simulink model "Main"  (R2022a)
settings: Solver=VariableStepAuto  StartTime=0.0  StopTime=30  RelTol=1e-3
values from neighbouring files (symbols this model uses):
  A_eq = double(A_eq)    [source_export.m]
  b = 7.66e-5    (= 7.66e-05)    [source_export.m]
  B_eq = double(B_eq)    [source_export.m]
  C = [1 0 0 0 0 0 0 0 0 0 0 0 ... (first row only)    [source_export.m]
  C_eq = C_final([1 2 3 6], 1:12)    [source_export.m]
  C_simulink = eye(12)    [source_export.m]
  Condition_0 = transpose([0 0 0 0 0 0 0 0 0 0 0 0])    [source_export.m]
  Condition_1 = transpose([0.2 0.2 0.2 0.2 0.2 0.2 0.2 0.2 0.2 0.2 0.2 0.2])    [source_export.m]
  D = zeros(4,4)    [source_export.m]
  d = 5.63e-6    (= 5.63e-06)    [source_export.m]
  D_Simulink = zeros(12,4)    [source_export.m]
  F = [      -20,   -20,   -20,   -21,   -21,   15,   -21.5, -21.5 ... (first row only)    [source_export.m]
  g = 9.81    [source_export.m]
  inv_G0 = inv_G_0( : , [1 , 2 ,3 ,6])    [source_export.m]
  inv_G0_LQR = inv_G_0_LQR( : , [1 , 2 ,3 ,6])    [source_export.m]
  Ixx = 8.5532e-3    (= 0.0085532)    [source_export.m]
  Iyy = 8.5532e-3    (= 0.0085532)    [source_export.m]
  Izz = 1.476e-2    (= 0.01476)    [source_export.m]
  K_d_LQR = K_LQR(:,1:12)    [source_export.m]
  K_q_LQR = K_LQR(:,12+1:12+4)    [source_export.m]
  Kfeedback = place(A_eq,B_eq,Poles)    [source_export.m]
  L = place(A_eq.',C_eq.',poles_obsv).'    [source_export.m]
  l = 0.22    [source_export.m]
  L_RO = 100*[1 2 1 14 ... (first row only)    [source_export.m]
  m = 1    [source_export.m]
  Q_1 = inv_mat2(:,1:q)    [source_export.m]
  Q_2 = inv_mat2(:,q+1:n)    [source_export.m]
  T_O = lyap(-F,A_eq,-L_RO*C)    [source_export.m]
undefined symbols (not defined in the file or in its folder): Discrete, K_LQR1, Time
libraries: slpidlib x8, simulink x6, ctrlSharedLib x1, sim3dlib x1, uavsim3dlib x1
(part 1 of 2)
settings Model: Creator=ali14  LastModifiedBy=ali14
settings ModelReferenceCC: EnableRefExpFcnMdlSchedulingChecks=off
settings RTWCC: Description=Generic Real-Time Target

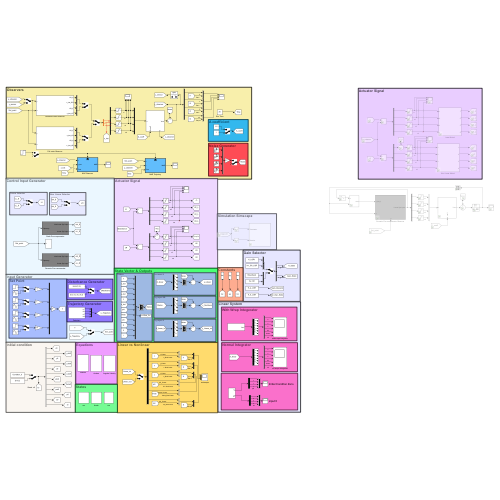
[thumbnail: Simulink's stored preview of the top-level diagram]
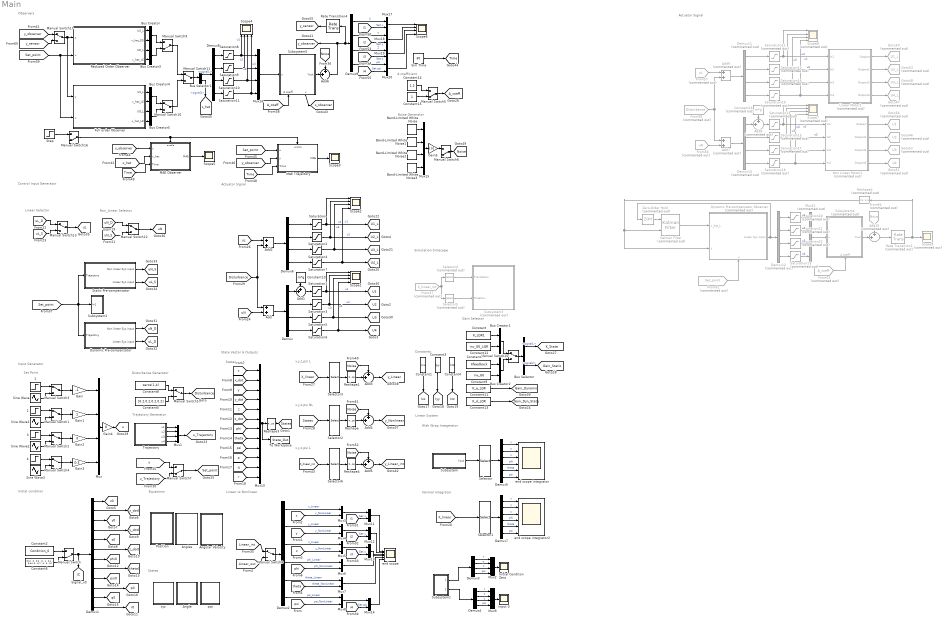
== system Main ==
  note: Observers
  note: A coefficient
  note: Noise Generator
  note: Gain Selector
  note: Actuator Signal
  note: States
  note: x,y,z,psi NL
  note: x,y,z,psi L
  note: Normal Integrator
  note: Trajectory Generator
  note: Linear Selector
  note: Non_Linear Selector
  note: Set Point
  note: Disturbance Generator
  note: State Vector & Outputs
  note: With Wrap Integerator
  note: Linear System
  note: Linear vs Nonlinear
  note: Constants
  note: Initial condition
  note: States
  note: Equations
  note: Input Generator
  note: Control Input Generator
  note: x,y,z,psi L
  note: Simulation Simscape
  note: Actuator Signal
  1 : Step  Time=3  SampleTime=0
  2 : Step  Time=3  SampleTime=0
  3 : Step  Time=0  SampleTime=0
  4 : Step  Time=5  SampleTime=0
  Add : Sum
  Add{1,3..6} (5 alike) : Sum  Inputs=++|
  Add10 : Sum  Commented=on  Inputs=++|
  Add2 : Sum
  Add7 : Sum  Commented=on
  Add8 : Sum  Commented=on  Inputs=++|
  Add9 : Sum  Commented=on
  Angle : Subsystem
  Angles : Subsystem
  Angular Velocity : Subsystem
  Band-Limited White Noise : simulink/Sources/Band-Limited White Noise  Cov=[0.000001]  Ts=0.01  seed=[23341]
  Band-Limited White Noise1 : simulink/Sources/Band-Limited White Noise  Cov=[0.000001]  Ts=0.1  seed=[23341]
  Band-Limited White Noise2 : simulink/Sources/Band-Limited White Noise  Cov=[0.0001]  Ts=0.1  seed=[23341]
  Band-Limited White Noise3 : simulink/Sources/Band-Limited White Noise  Cov=[0.00001]  Ts=0.1  seed=[23341]
  Bus Creator{,1..5} (6 alike) : BusCreator  Inputs=2
  Bus Selector : BusSelector  OutputSignals=signal1,signal2
  Bus Selector1 : BusSelector  OutputSignals=signal1,signal2
  Constant : Constant  Value=K_LQR1
  Constant1 : Constant  Value=Ixx
  Constant10 : Constant  Value=m*g
  Constant11 : Constant  Value=K_q_LQR
  Constant12 : Constant  Value=inv_G0_LQR
  Constant13 : Constant  Value=K_d_LQR
  Constant14 : Constant  Value=1.2
  Constant15 : Constant
  Constant16 : Constant  Commented=on  Value=m*g
  Constant2 : Constant  Value=Condition_0
  Constant3 : Constant  Value=Iyy
  Constant4 : Constant  Value=Izz
  Constant5 : Constant  Value=[0.2,0.2,0.2,0.2]
  Constant6 : Constant  Value=[0.2 , 0 , 0.2 , 0 , 1 , 0.4 , 0.04 ,0 , 0.7 , 0 , 0 , 0]
  Constant7 : Constant  Value=Kfeedback
  Constant8 : Constant  Value=zeros(1,4)
  Constant9 : Constant  Value=inv_G0
  Demux{,3..4,6,8..9} (6 alike) : Demux
  Demux1 : Demux  Outputs=12
  Demux10 : Demux  Commented=on
  Demux11 : Demux  Commented=on
  Demux12 : Demux  Commented=on
  Demux2 : Demux  Outputs=6
  Demux5 : Demux  Outputs=6
  Demux7 : Demux  Outputs=6
  Dynamic Pre-compensator : Subsystem
  Dynamic Pre-compensator Observer : Subsystem  Commented=on
      settings: PortSchema="{\"entries\":[{\"content\":{\"sides\":[{\"content\":{\"connectorIds\":[\"In1\",\"In2\"]},\"type\":\"ConnectorPlacement.EquallySpacedRectSide\",\"uuid\":\"7ff58fb8-8d2b-4c8e-a591-1a745530a661\"},{\"content\":{\"connectorIds\":[\"Out1\"],\"side\":\"RIGHT\"},\"type\":\"ConnectorPlacement.EquallySpacedRectSide\",\"uuid\":\"18d93ec8-0d87-4739-af88-4b64d8e2703a\"},{\"content\":{\"connectorIds\":[],\"side\":\"TOP\"},\"type\":\"ConnectorPlacement.EquallySpacedRectSide\",\"uuid\":\"fcb1c7ab-ae0a-4067-b3dc-1c5dc69aae1f\"},{\"content\":{\"connectorIds\":[\"In3\"],\"side\":\"BOTTOM\"},\"type\":\"ConnectorPlacement.EquallySpacedRectSide\",\"uuid\":\"838d79c5-32f8-45c9-a35f-55d5e51129e3\"}]},\"type\":\"ConnectorPlacement.EquallySpacedConnector\",\"uuid\":\"97c2476e-220b-403a-9339-6beb5ac026c2\"}],\"packageUris\":[\"http://schema.mathworks.com/mf0/Connector/R2020b\"],\"version\":\"1.0\"}"
  From47 : From  Commented=on  GotoTag=X_linear_int  TagVisibility=global
  From56 : From  Commented=on  GotoTag=uN  TagVisibility=global
  From57 : From  Commented=on  GotoTag=uL  TagVisibility=global
  From58 : From  Commented=on  GotoTag=Disturbance  TagVisibility=global
  From62 : From  Commented=on  GotoTag=Set_point  TagVisibility=global
  From63 : From  Commented=on  GotoTag=A_coeff  TagVisibility=global
  From64 : From  Commented=on  GotoTag=Noise  TagVisibility=global
  Full order Observer : Subsystem
  Gain : Gain  Gain=-1
  Gain1 : Gain
  Gain2 : Gain  Gain=3
  Gain3 : Gain  Gain=0.3
  Gain4 : Gain  Gain=0
  Gain5 : Gain  Gain=0.01
  Goto46 : Goto  Commented=on  GotoTag=U2  TagVisibility=global
  Goto47 : Goto  Commented=on  GotoTag=U4_L  TagVisibility=global
  Goto48 : Goto  Commented=on  GotoTag=U3_L  TagVisibility=global
  Goto50 : Goto  Commented=on  GotoTag=U1_L  TagVisibility=global
  Goto51 : Goto  Commented=on  GotoTag=U4  TagVisibility=global
  Goto52 : Goto  Commented=on  GotoTag=U3  TagVisibility=global
  Goto53 : Goto  Commented=on  GotoTag=U2_L  TagVisibility=global
  Goto54 : Goto  Commented=on  GotoTag=U1  TagVisibility=global
  Initial Conditon Zero : Scope
  Kalman Filter : ctrlSharedLib/Kalman Filter  Commented=on  TimeDomain=Discrete-Time  UseCurrentEstimator=on  ModelSource=Individual A, B, C, D matrices  ModelSourceVariable=ss(0.95,1,1,0,1)  A=A_eq  B=B_eq  C=C_eq  D=D  NumberOfStates=12  NumberOfInputs=4  NumberOfOutputs=4  InitialEstimateSource=Dialog  X0=0  P0=10  UseK=off  UseGH=off  NumberOfProcessNoiseInputs=1  G=1  TimeInvariantG=on  H=0  TimeInvariantH=on  Q=0.05  TimeInvariantQ=on  R=1  TimeInvariantR=on  N=0  TimeInvariantN=on  AddInputPort=on  AddEnablePort=off  OutputEstimatedY=off  OutputP=off  Ts=-1
  Linear Motor1 : Subsystem  Commented=on
  MAE Observer : Subsystem
  MAE Trajectory : Subsystem
  Manual Switch{,5..7,9,16} (6 alike) : ManualSwitch  CurrentSetting=0
  Manual Switch{1..4,8,10..15,17} (12 alike) : ManualSwitch
  Mux{,1..2,9,15..16} (6 alike) : Mux
  Mux10 : Mux  Inputs=12
  Mux{3..8,11..14,17..20} (14 alike) : Mux  Inputs=2
  Mux21 : Mux  Commented=on
  Non Linear Motor1 : Subsystem  Commented=on
  Position : Subsystem
  Rate Transition1 : RateTransition  Commented=on  OutPortSampleTime=0.01
  Rate Transition4 : RateTransition  OutPortSampleTime=0.01
  Reduced Order Observer : Subsystem
  Reshape{,1,3..4} (4 alike) : Reshape  OutputDimensionality=Column vector (2-D)
  Reshape2 : Reshape  Commented=on  OutputDimensionality=Column vector (2-D)
  Saturation : Saturate  UpperLimit=15  LowerLimit=-10
  Saturation1 : Saturate  UpperLimit=25  LowerLimit=0
  Saturation{2..5,9..10} (6 alike) : Saturate  UpperLimit=1.5  LowerLimit=-1.5
  Saturation11 : Saturate  UpperLimit=1  LowerLimit=-1
  Saturation12 : Saturate  Commented=on  UpperLimit=15  LowerLimit=-10
  Saturation13 : Saturate  Commented=on  UpperLimit=25  LowerLimit=0
  Saturation{14..17,21..22} (6 alike) : Saturate  Commented=on  UpperLimit=1.5  LowerLimit=-1.5
  Saturation18 : Saturate  Commented=on  UpperLimit=1  LowerLimit=-1
  Saturation19 : Saturate  Commented=on  UpperLimit=1  LowerLimit=-1
  Saturation20 : Saturate  Commented=on  UpperLimit=15  LowerLimit=-10
  Saturation23 : Saturate  Commented=on  UpperLimit=1  LowerLimit=-1
  Saturation6 : Saturate  UpperLimit=1  LowerLimit=-1
  Saturation7 : Saturate  UpperLimit=1  LowerLimit=-1
  Saturation8 : Saturate  UpperLimit=15  LowerLimit=-10
  Scope{1..2,4,6} (4 alike) : Scope  NumInputPorts=4
  Scope3 : Scope
  Scope5 : Scope
  Scope7 : Scope  Commented=on  NumInputPorts=4
  Scope8 : Scope  Commented=on  NumInputPorts=4
  Scope9 : Scope  Commented=on
  Selector : Selector  InputPortWidth=12  IndexOptions=Index vector (dialog)  Indices=[1 3 5 7 8 9]  OutputSizes=1
  Selector1 : Selector  InputPortWidth=12  IndexOptions=Index vector (dialog)  Indices=[1 3 5 7 8 9]  OutputSizes=1
  Selector2 : Selector  InputPortWidth=12  IndexOptions=Index vector (dialog)  Indices=[1 3 5 9]  OutputSizes=1
  Selector3 : Selector  InputPortWidth=12  IndexOptions=Index vector (dialog)  Indices=[1 3 5 9]  OutputSizes=1
  Selector4 : Selector  Commented=on  InputPortWidth=12  IndexOptions=Index vector (dialog)  Indices=[1 3 5]  OutputSizes=1
  Selector5 : Selector  Commented=on  InputPortWidth=12  IndexOptions=Index vector (dialog)  Indices=[9 7 8 ]  OutputSizes=1
  Selector6 : Selector  InputPortWidth=12  IndexOptions=Index vector (dialog)  Indices=[1 3 5 9]  OutputSizes=1
  Sim TIme : Constant  Value=30
  Sine Wave{,1..3} (4 alike) : Sin  SampleTime=0
  Static Pre-compensator : Subsystem
  Step : Step  Time=0  SampleTime=0
  Subsystem : Subsystem
  Subsystem1 : Subsystem
  Subsystem2 : Subsystem
  Subsystem3 : Subsystem  Commented=on
  Subsystem4 : Subsystem  Commented=on
      settings: PortSchema="{\"entries\":[{\"content\":{\"sides\":[{\"content\":{\"connectorIds\":[\"In1\"]},\"type\":\"ConnectorPlacement.EquallySpacedRectSide\",\"uuid\":\"35a88aa3-78e6-4d31-af9d-f5149068514e\"},{\"content\":{\"connectorIds\":[\"Out1\"],\"side\":\"RIGHT\"},\"type\":\"ConnectorPlacement.EquallySpacedRectSide\",\"uuid\":\"0f0b60d9-c9a7-4a63-831d-7f164469e2c4\"},{\"content\":{\"connectorIds\":[],\"side\":\"TOP\"},\"type\":\"ConnectorPlacement.EquallySpacedRectSide\",\"uuid\":\"a6909642-0e23-4ad5-9187-38e4eb793ad9\"},{\"content\":{\"connectorIds\":[\"In2\"],\"side\":\"BOTTOM\"},\"type\":\"ConnectorPlacement.EquallySpacedRectSide\",\"uuid\":\"6bcb8c31-d0ff-4cff-a0ca-573413c8c784\"}]},\"type\":\"ConnectorPlacement.EquallySpacedConnector\",\"uuid\":\"6b3745e7-cbc0-4f87-a93b-0b31a1f6abb0\"}],\"packageUris\":[\"http://schema.mathworks.com/mf0/Connector/R2020b\"],\"version\":\"1.0\"}"
  Subsystem5 : Subsystem
      settings: PortSchema="{\"entries\":[{\"content\":{\"sides\":[{\"content\":{\"connectorIds\":[\"In1\"]},\"type\":\"ConnectorPlacement.EquallySpacedRectSide\",\"uuid\":\"35a88aa3-78e6-4d31-af9d-f5149068514e\"},{\"content\":{\"connectorIds\":[\"Out1\"],\"side\":\"RIGHT\"},\"type\":\"ConnectorPlacement.EquallySpacedRectSide\",\"uuid\":\"0f0b60d9-c9a7-4a63-831d-7f164469e2c4\"},{\"content\":{\"connectorIds\":[],\"side\":\"TOP\"},\"type\":\"ConnectorPlacement.EquallySpacedRectSide\",\"uuid\":\"a6909642-0e23-4ad5-9187-38e4eb793ad9\"},{\"content\":{\"connectorIds\":[\"In2\",\"Out2\"],\"side\":\"BOTTOM\"},\"type\":\"ConnectorPlacement.EquallySpacedRectSide\",\"uuid\":\"6bcb8c31-d0ff-4cff-a0ca-573413c8c784\"}]},\"type\":\"ConnectorPlacement.EquallySpacedConnector\",\"uuid\":\"6b3745e7-cbc0-4f87-a93b-0b31a1f6abb0\"}],\"packageUris\":[\"http://schema.mathworks.com/mf0/Connector/R2020b\"],\"version\":\"1.0\"}"
  To Workspace : ToWorkspace  VariableName=State_Out  SampleTime=-1
  "Trajectory " : Subsystem
  Zero-Order Hold : ZeroOrderHold  Commented=on  SampleTime=0.01
  end scope : Scope  NumInputPorts=6
  end scope integrator : Scope  NumInputPorts=6
  end scope integrator2 : Scope  NumInputPorts=6
  input 0 : Scope
  pqr : Subsystem
  xyz : Subsystem
  tag scope: A_coeff=global, Disturbance=global, Gain_Dyn_State=global, Gain_Dynamic=global, Gain_Static=global, IC=global, Ixx=global, Iyy=global, Izz=global, K_State=global, Noise=global, Set_point=global, States=global, Time=global, U1=global, U1_L=global, U2=global, U2_L=global, U3=global, U3_L=global, U4=global, U4_L=global, p0=global, phi0=global, psi0=global, q0=global, r0=global, theta0=global, u=global, uL=global, uL_D=global, uL_S=global, uN=global, uN_D=global, uN_S=global, u_Trajectory=global, x0=global, x_dot0=global, x_hat=global, x_observer=global, y0=global, y_Linear=global, y_Linear_int=global, y_Nonlinear=global, y_dot0=global, y_observer=global, y_sensor=global, z0=global, z_dot0=global
  wires:
  Demux1/1 -> [x0]
  Demux1/3 -> [y0]
  Demux1/5 -> [z0]
  Demux1/2 -> [x_dot0]
  Demux1/4 -> [y_dot0]
  Demux1/6 -> [z_dot0]
  Demux1/7 -> [phi0]
  Demux1/8 -> [theta0]
  Demux1/9 -> [psi0]
  Demux1/10 -> [p0]
  Demux1/11 -> [q0]
  Demux1/12 -> [r0]
  Constant1/1 -> [Ixx]
  Constant3/1 -> [Iyy]
  Constant4/1 -> [Izz]
  Constant6/1 -> Manual Switch/2
  Manual Switch/1 -> Demux1/1, [IC]
  Constant2/1 -> Manual Switch/1
  Demux2/1 -> Mux3/1  "x_Linear"
  [x] -> Mux3/2  "x_NonLinear"
  Demux2/2 -> Mux4/1  "y_Linear"
  Demux2/3 -> Mux5/1  "z_Linear"
  Demux2/4 -> Mux6/1  "phi_Linear"
  Demux2/5 -> Mux7/1  "theta_Linear"
  Demux2/6 -> Mux8/1  "psi_Linear"
  [y] -> Mux4/2  "y_NonLinear"
  [z] -> Mux5/2  "z_NonLinear"
  [phi] -> Mux6/2  "phi_NonLinear"
  [psi] -> Mux8/2  "psi_NonLinear"
  [theta] -> Mux7/2  "theta_NonLinear"
  Mux6/1 -> end scope/4
  Mux7/1 -> end scope/5
  Subsystem1/1(Outport) -> Demux3/1
  Demux3/1 -> Mux2/1  "x"
  Demux3/2 -> Mux2/2  "y"
  Demux3/3 -> Mux2/3  "z"
  Demux3/4 -> Mux2/4  "psi"
  Mux2/1 -> Initial Conditon Zero/1
  Demux4/2 -> Mux9/2  "y"
  Demux4/1 -> Mux9/1  "x"
  Demux4/4 -> Mux9/4  "psi"
  Demux4/3 -> Mux9/3  "z"
  Subsystem1/2(Outport1) -> Demux4/1
  Mux9/1 -> input 0/1
  Subsystem/1(Yout) -> Selector/1
  Selector/1 -> Demux5/1
  Demux5/1 -> end scope integrator/1  "x"
  Demux5/2 -> end scope integrator/2  "y"
  Demux5/3 -> end scope integrator/3  "z"
  Demux5/4 -> end scope integrator/4  "phi"
  Demux5/5 -> end scope integrator/5  "theta"
  Demux5/6 -> end scope integrator/6  "psi"
  [x] -> Mux10/1
  [x_dot] -> Mux10/2
  [y] -> Mux10/3
  [y_dot] -> Mux10/4
  [z] -> Mux10/5
  [z_dot] -> Mux10/6
  [phi] -> Mux10/7
  [theta] -> Mux10/8
  [psi] -> Mux10/9
  [p] -> Mux10/10
  [q] -> Mux10/11
  [r] -> Mux10/12
  3/1 -> Manual Switch2/1
  Gain2/1 -> Mux/3
  1/1 -> Manual Switch3/1
  Manual Switch4/1 -> Gain3/1
  Manual Switch2/1 -> Gain2/1
  Sine Wave2/1 -> Manual Switch2/2
  Gain3/1 -> Mux/4
  4/1 -> Manual Switch4/1
  Sine Wave3/1 -> Manual Switch4/2
  Sine Wave/1 -> Manual Switch3/2
  Gain/1 -> Mux/1
  Gain1/1 -> Mux/2
  Sine Wave1/1 -> Manual Switch1/2
  2/1 -> Manual Switch1/1
  Manual Switch1/1 -> Gain1/1
  Demux7/2 -> end scope integrator2/2  "y"
  Demux7/6 -> end scope integrator2/6  "psi"
  Demux7/4 -> end scope integrator2/4  "phi"
  [X_linear] -> Selector1/1
  Demux7/3 -> end scope integrator2/3  "z"
  Demux7/5 -> end scope integrator2/5  "theta"
  Selector1/1 -> Demux7/1
  Demux7/1 -> end scope integrator2/1  "x"
  Manual Switch14/1 -> [Disturbance]
  Constant8/1 -> Manual Switch14/1
  Constant5/1 -> Manual Switch14/2
  Bus Selector/1 -> [K_State]  "<signal1>"
  Demux6/1 -> Saturation/1
  Demux6/3 -> Saturation4/1
  Demux6/2 -> Saturation2/1
  Demux6/4 -> Saturation7/1
  Demux/1 -> Add1/2
  Demux/4 -> Saturation6/1
  Demux/3 -> Saturation5/1
  Constant10/1 -> Add1/1
  Demux/2 -> Saturation3/1
  Add1/1 -> Saturation1/1
  Static Pre-compensator/2(Linear Sys input) -> [uL_S]
  Static Pre-compensator/1(Non linear Sys input) -> [uN_S]
  Dynamic Pre-compensator/2(Linear Sys input) -> [uL_D]
  Dynamic Pre-compensator/1(Non linear Sys input) -> [uN_D]
  Selector3/1 -> Reshape1/1
  Selector2/1 -> Reshape/1
  [X_linear] -> Selector3/1
  Mux10/1 -> Reshape3/1, To Workspace/1
  [States] -> Selector2/1
  [uN] -> Add/2
  [Disturbance] -> Add2/2, Add/1
  Add2/1 -> Demux6/1
  Add/1 -> Demux/1
  [uL] -> Add2/1
  Constant/1 -> Bus Creator1/1
  Constant12/1 -> Bus Creator1/2
  Constant7/1 -> Bus Creator2/1
  Constant9/1 -> Bus Creator2/2
  Bus Creator1/1 -> Manual Switch15/1
  Bus Creator2/1 -> Manual Switch15/2
  Manual Switch15/1 -> Bus Selector/1
  Bus Selector/2 -> [Gain_Static]  "<signal2>"
  "Trajectory "/4(u4) -> Mux1/4
  Mux1/1 -> [u_Trajectory]
  "Trajectory "/1(u1) -> Mux1/1
  "Trajectory "/2(u2) -> Mux1/2
  "Trajectory "/3(u3) -> Mux1/3
  Mux3/1 -> Mux11/1
  [i1] -> Mux11/2  "Set x"
  Mux11/1 -> end scope/1
  [i2] -> Mux12/2  "Set y"
  Mux4/1 -> Mux12/1
  Mux12/1 -> end scope/2
  [i3] -> Mux13/2  "Set z"
  Mux5/1 -> Mux13/1
  Mux13/1 -> end scope/3
  [i4] -> Mux14/2  "Set psi"
  Mux8/1 -> Mux14/1
  Mux14/1 -> end scope/6
  Manual Switch8/1 -> Demux2/1
  [Linear_out] -> Manual Switch8/2
  [Linear_int] -> Manual Switch8/1
  Manual Switch3/1 -> Gain/1
  Mux/1 -> Gain4/1
  Gain4/1 -> [u]
  Constant11/1 -> [Gain_Dynamic]
  Constant13/1 -> [Gain_Dyn_State]
  [u_Trajectory] -> Manual Switch7/2
  [u] -> Manual Switch7/1
  [Set_point] -> Dynamic Pre-compensator/1(Trajectory), Subsystem2/1(In1), Static Pre-compensator/1(Trajectory)
  Reshape3/1 -> [States]
  Manual Switch7/1 -> [Set_point]
  [X_linear_int] -> Selector6/1
  Selector6/1 -> Reshape4/1
  Saturation/1 -> [U1_L], Scope2/1  "u1"
  Saturation1/1 -> [U1], Scope1/1  "u1"
  Saturation2/1 -> [U2_L], Scope2/2  "u2"
  Saturation3/1 -> [U2], Scope1/2  "u2"
  Saturation4/1 -> [U3_L], Scope2/3  "u3"
  Saturation5/1 -> [U3], Scope1/3  "u3"
  Saturation6/1 -> [U4], Scope1/4  "u4"
  Saturation7/1 -> [U4_L], Scope2/4  "u4"
  [Set_point] -> Reduced Order Observer/2(u), Full order Observer/2(u)
  Band-Limited White Noise/1 -> Mux15/1
  Band-Limited White Noise1/1 -> Mux15/2
  Band-Limited White Noise2/1 -> Mux15/3
  Band-Limited White Noise3/1 -> Mux15/4
  Reshape1/1 -> Add3/2
  Add3/1 -> [y_Linear]
  [Noise] -> Add3/1
  Reshape/1 -> Add4/2
  Add4/1 -> [y_Nonlinear]
  [Noise] -> Add4/1
  Reshape4/1 -> Add5/2
  Add5/1 -> [y_Linear_int]
  [Noise] -> Add5/1
  Manual Switch6/1 -> [Noise]
  Saturation11/1 -> Mux16/4, Scope4/4  "u4"
  Saturation8/1 -> Mux16/1, Scope4/1  "u1"
  Demux8/1 -> Saturation8/1
  Saturation10/1 -> Mux16/3, Scope4/3  "u3"
  Saturation9/1 -> Mux16/2, Scope4/2  "u2"
  Demux8/2 -> Saturation9/1
  Demux8/3 -> Saturation10/1
  Demux8/4 -> Saturation11/1
  Mux16/1 -> Subsystem5/1(u)
  Reduced Order Observer/4(x_hat_LS) -> Bus Creator3/2
  Subsystem5/1(Yout) -> Add6/2
  Add6/1 -> [y_observer], Rate Transition4/1, Demux9/1
  [Noise] -> Add6/1
  Constant14/1 -> Manual Switch5/1
  Constant15/1 -> Manual Switch5/2
  MAE Observer/1(MAE) -> Scope5/1
  Demux9/1 -> Mux17/1  "X"
  Demux9/3 -> Mux19/1  "Z"
  Demux9/2 -> Mux18/1  "Y"
  Demux9/4 -> Mux20/1  "psi"
  Mux15/1 -> Gain5/1
  Gain5/1 -> Manual Switch6/1
  Reduced Order Observer/2(x_hat_DS) -> Bus Creator/2
  Reduced Order Observer/1(US_L) -> Bus Creator/1
  Manual Switch11/1 -> Bus Selector1/1
  Reduced Order Observer/3(UD_L) -> Bus Creator3/1
  Full order Observer/1(US_L) -> Bus Creator4/1
  Full order Observer/2(x_hat_LS) -> Bus Creator4/2
  Full order Observer/3(UD_L) -> Bus Creator5/1
  Full order Observer/4(x_hat_LD) -> Bus Creator5/2
  Bus Creator/1 -> Manual Switch9/1
  Bus Creator3/1 -> Manual Switch9/2
  Bus Creator4/1 -> Manual Switch10/1
  Bus Creator5/1 -> Manual Switch10/2
  Manual Switch9/1 -> Manual Switch11/1
  Manual Switch10/1 -> Manual Switch11/2
  [uN_D] -> Manual Switch12/1
  [uN_S] -> Manual Switch12/2
  Manual Switch12/1 -> [uN]
  Manual Switch13/1 -> [uL]
  [uL_D] -> Manual Switch13/1
  [uL_S] -> Manual Switch13/2
  Manual Switch5/1 -> [A_coeff]
  [A_coeff] -> Subsystem5/2(A coeff)
  Subsystem5/2(x) -> [x_observer]
  Bus Selector1/1 -> Demux8/1  "<signal1>"
  Bus Selector1/2 -> [x_hat]  "<signal2>"
  [x_observer] -> MAE Observer/1(x)
  [x_hat] -> MAE Observer/2(x_hat)
  [Set_point] -> MAE Trajectory/1(u)
  [y_observer] -> MAE Trajectory/2(y)
  MAE Trajectory/1(MAE) -> Scope3/1
  Sim TIme/1 -> [Time]
  From47/1 -> Selector4/1, Selector5/1
  [Time] -> MAE Trajectory/3(Time)
  [Time] -> MAE Observer/3(Time)
  Step/1 -> Manual Switch16/1
  Manual Switch16/1 -> MAE Observer/Enable, MAE Trajectory/Enable
  [i1] -> Mux17/2  "Set x"
  Mux17/1 -> Scope6/1
  [i2] -> Mux18/2  "Set y"
  [i3] -> Mux19/2  "Set z"
  [i4] -> Mux20/2  "Set psi"
  Mux18/1 -> Scope6/2
  Mux19/1 -> Scope6/3
  Mux20/1 -> Scope6/4
  Selector4/1 -> Subsystem3/1(Translation)
  Selector5/1 -> Subsystem3/2(Rotation)
  Non Linear Motor1/4(Outport3) -> Goto51/1
  Saturation14/1 -> Linear Motor1/2(In2), Scope8/2  "u2"
  Add9/1 -> Demux11/1
  Linear Motor1/4(Outport3) -> Goto47/1
  From57/1 -> Add9/1
  Demux10/3 -> Saturation17/1
  Add7/1 -> Demux10/1
  Linear Motor1/2(Outport1) -> Goto53/1
  From56/1 -> Add7/2
  Demux11/1 -> Saturation12/1
  Demux10/4 -> Saturation18/1
  Constant16/1 -> Add8/1
  Demux10/2 -> Saturation15/1
  Linear Motor1/3(Outport2) -> Goto48/1
  Demux11/4 -> Saturation19/1
  Demux11/3 -> Saturation16/1
  Saturation18/1 -> Non Linear Motor1/4(In4), Scope7/4  "u4"
  Demux10/1 -> Add8/2
  Saturation16/1 -> Scope8/3, Linear Motor1/3(In3)  "u3"
  Saturation13/1 -> Non Linear Motor1/1(In1), Scope7/1  "u1"
  Non Linear Motor1/1(Outport) -> Goto54/1
  Saturation17/1 -> Non Linear Motor1/3(In3), Scope7/3  "u3"
  Saturation19/1 -> Linear Motor1/4(In4), Scope8/4  "u4"
  Non Linear Motor1/3(Outport2) -> Goto52/1
  Linear Motor1/1(Outport) -> Goto50/1
  Saturation15/1 -> Non Linear Motor1/2(In2), Scope7/2  "u2"
  Saturation12/1 -> Linear Motor1/1(In1), Scope8/1  "u1"
  From58/1 -> Add9/2, Add7/1
  Add8/1 -> Saturation13/1
  Demux11/2 -> Saturation14/1
  Non Linear Motor1/2(Outport1) -> Goto46/1
  Manual Switch17/1 -> Full order Observer/1(y), Reduced Order Observer/1(y)
  [y_observer] -> Manual Switch17/1
  [y_sensor] -> Manual Switch17/2
  Rate Transition4/1 -> [y_sensor]
  Rate Transition1/1 -> Scope9/1, Reshape2/1
  Kalman Filter/1 -> Dynamic Pre-compensator Observer/1(x_hat_L)
  From62/1 -> Dynamic Pre-compensator Observer/3(u)
  Demux12/3 -> Saturation22/1
  Demux12/2 -> Saturation21/1
  Demux12/4 -> Saturation23/1
  Demux12/1 -> Saturation20/1
  Dynamic Pre-compensator Observer/1(Linear Sys input) -> Zero-Order Hold/1, Demux12/1
  Saturation20/1 -> Mux21/1  "u1"
  Saturation21/1 -> Mux21/2  "u2"
  Saturation22/1 -> Mux21/3  "u3"
  Saturation23/1 -> Mux21/4  "u4"
  Mux21/1 -> Subsystem4/1(u)
  From63/1 -> Subsystem4/2(A coeff)
  From64/1 -> Add10/1
  Subsystem4/1(Yout) -> Add10/2
  Add10/1 -> Rate Transition1/1
  Reshape2/1 -> Kalman Filter/2, Dynamic Pre-compensator Observer/2(y)
  Zero-Order Hold/1 -> Kalman Filter/1

== system Main/Angle ==
  Integrator1 : Integrator  InitialConditionSource=external  WrapState=on
  Integrator2 : Integrator  InitialConditionSource=external  WrapState=on
  Integrator3 : Integrator  InitialConditionSource=external  WrapState=on
  tag scope: phi=global, psi=global, theta=global
  wires:
  Integrator2/1 -> [theta]
  [theta_dot] -> Integrator2/1
  Integrator3/1 -> [psi]
  [theta0] -> Integrator2/2
  [psi_dot] -> Integrator3/1
  [phi0] -> Integrator1/2
  Integrator1/1 -> [phi]
  [psi0] -> Integrator3/2
  [phi_dot] -> Integrator1/1

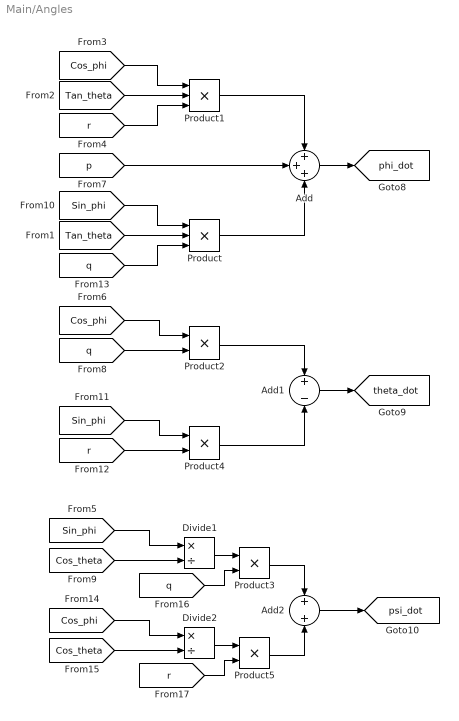
== system Main/Angles ==
  Add : Sum  Inputs=+++
  Add1 : Sum  Inputs=+-
  Add2 : Sum
  Divide1 : Product  Inputs=*/
  Divide2 : Product  Inputs=*/
  Product : Product  Inputs=3
  Product1 : Product  Inputs=3
  Product{2..5} (4 alike) : Product
  tag scope: phi_dot=global, psi_dot=global, theta_dot=global
  wires:
  [Sin_phi] -> Product/1
  [Tan_theta] -> Product/2
  [q] -> Product/3
  Product/1 -> Add/3
  [p] -> Add/2
  [Cos_phi] -> Product1/1
  [Tan_theta] -> Product1/2
  [r] -> Product1/3
  Product1/1 -> Add/1
  Add/1 -> [phi_dot]
  Add1/1 -> [theta_dot]
  [Cos_phi] -> Product2/1
  [q] -> Product2/2
  Product2/1 -> Add1/1
  Product4/1 -> Add1/2
  [Sin_phi] -> Divide1/1
  [Cos_theta] -> Divide1/2
  Divide1/1 -> Product3/1
  [r] -> Product4/2
  [Sin_phi] -> Product4/1
  Add2/1 -> [psi_dot]
  Product3/1 -> Add2/1
  [Cos_phi] -> Divide2/1
  Divide2/1 -> Product5/1
  [Cos_theta] -> Divide2/2
  Product5/1 -> Add2/2
  [q] -> Product3/2
  [r] -> Product5/2

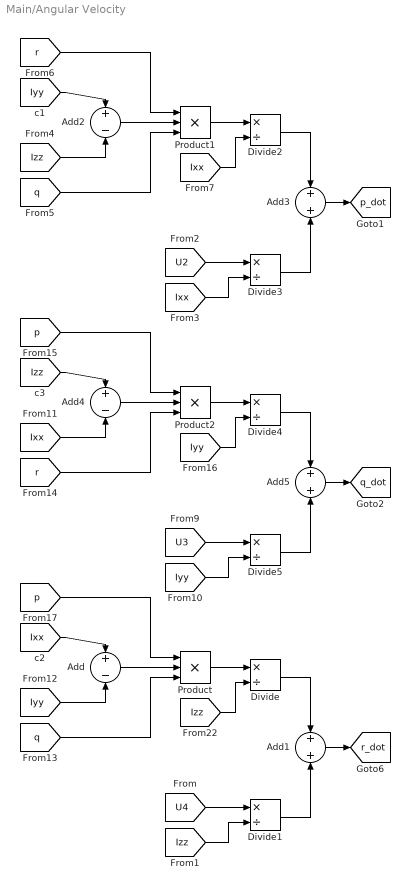
== system Main/Angular Velocity ==
  Add : Sum  Inputs=+-
  Add1 : Sum
  Add2 : Sum  Inputs=+-
  Add3 : Sum
  Add4 : Sum  Inputs=+-
  Add5 : Sum
  Divide{,1..5} (6 alike) : Product  Inputs=*/
  Product : Product  Inputs=3
  Product1 : Product  Inputs=3
  Product2 : Product  Inputs=3
  tag scope: p_dot=global, q_dot=global, r_dot=global
  wires:
  [Ixx] -> Add/1
  [Iyy] -> Add/2
  Add/1 -> Product/2
  [p] -> Product/1
  [q] -> Product/3
  Product/1 -> Divide/1
  [Izz] -> Divide/2
  Divide/1 -> Add1/1
  Add1/1 -> [r_dot]
  [U4] -> Divide1/1
  [Izz] -> Divide1/2
  Divide1/1 -> Add1/2
  [Izz] -> Add2/2
  Add2/1 -> Product1/2
  [r] -> Product1/1
  [U2] -> Divide3/1
  Add3/1 -> [p_dot]
  Divide2/1 -> Add3/1
  [Ixx] -> Divide3/2
  [q] -> Product1/3
  [Ixx] -> Divide2/2
  Product1/1 -> Divide2/1
  [Iyy] -> Add2/1
  Divide3/1 -> Add3/2
  [U3] -> Divide5/1
  [Iyy] -> Divide4/2
  Add5/1 -> [q_dot]
  [Iyy] -> Divide5/2
  Product2/1 -> Divide4/1
  [p] -> Product2/1
  Divide4/1 -> Add5/1
  [r] -> Product2/3
  Divide5/1 -> Add5/2
  [Ixx] -> Add4/2
  [Izz] -> Add4/1
  Add4/1 -> Product2/2

== system Main/Dynamic Pre-compensator ==
  Trajectory : Inport
  Add : Sum  Inputs=+-
  Add1 : Sum  Inputs=-+
  Add2 : Sum  Inputs=--
  Add3 : Sum  Inputs=--
  Integrator : Integrator
  Integrator1 : Integrator
  Matrix Multiply{,1..3} (4 alike) : Product  Multiplication=Matrix(*)
  Non linear Sys input : Outport
  Linear Sys input : Outport  Port=2
  wires:
  Trajectory/1 -> Add1/2, Add/1
  [y_Linear_int] -> Add/2
  [y_Nonlinear] -> Add1/1
  Add1/1 -> Integrator/1
  Add/1 -> Integrator1/1
  Integrator1/1 -> Matrix Multiply1/2
  [Gain_Dynamic] -> Matrix Multiply/1, Matrix Multiply1/1
  [Gain_Dyn_State] -> Matrix Multiply3/1
  [States] -> Matrix Multiply2/2
  [Gain_Dyn_State] -> Matrix Multiply2/1
  [X_linear] -> Matrix Multiply3/2
  Matrix Multiply/1 -> Add2/2
  Matrix Multiply2/1 -> Add2/1
  Matrix Multiply1/1 -> Add3/1
  Matrix Multiply3/1 -> Add3/2
  Add2/1 -> Non linear Sys input/1
  Add3/1 -> Linear Sys input/1
  Integrator/1 -> Matrix Multiply/2

== system Main/Dynamic Pre-compensator Observer ==
  x_hat_L : Inport
  y : Inport  Port=2
  u : Inport  Port=3
  Add : Sum  Inputs=+-
  Add3 : Sum  Inputs=--
  Integrator1 : Integrator
  Matrix Multiply1 : Product  Multiplication=Matrix(*)
  Matrix Multiply3 : Product  Multiplication=Matrix(*)
  Linear Sys input : Outport
  wires:
  u/1 -> Add/1
  y/1 -> Add/2
  Add/1 -> Integrator1/1
  Integrator1/1 -> Matrix Multiply1/2
  [Gain_Dynamic] -> Matrix Multiply1/1
  [Gain_Dyn_State] -> Matrix Multiply3/1
  x_hat_L/1 -> Matrix Multiply3/2
  Matrix Multiply1/1 -> Add3/1
  Matrix Multiply3/1 -> Add3/2
  Add3/1 -> Linear Sys input/1

== system Main/Full order Observer ==
  note: Full order Observer
  y : Inport
  u : Inport  Port=2
  Dynamic Pre-compensator Observer : Subsystem
      settings: PortSchema="{\"entries\":[{\"content\":{\"sides\":[{\"content\":{\"connectorIds\":[\"In1\",\"In2\"]},\"type\":\"ConnectorPlacement.EquallySpacedRectSide\",\"uuid\":\"7ff58fb8-8d2b-4c8e-a591-1a745530a661\"},{\"content\":{\"connectorIds\":[\"Out1\"],\"side\":\"RIGHT\"},\"type\":\"ConnectorPlacement.EquallySpacedRectSide\",\"uuid\":\"18d93ec8-0d87-4739-af88-4b64d8e2703a\"},{\"content\":{\"connectorIds\":[],\"side\":\"TOP\"},\"type\":\"ConnectorPlacement.EquallySpacedRectSide\",\"uuid\":\"fcb1c7ab-ae0a-4067-b3dc-1c5dc69aae1f\"},{\"content\":{\"connectorIds\":[\"In3\"],\"side\":\"BOTTOM\"},\"type\":\"ConnectorPlacement.EquallySpacedRectSide\",\"uuid\":\"838d79c5-32f8-45c9-a35f-55d5e51129e3\"}]},\"type\":\"ConnectorPlacement.EquallySpacedConnector\",\"uuid\":\"97c2476e-220b-403a-9339-6beb5ac026c2\"}],\"packageUris\":[\"http://schema.mathworks.com/mf0/Connector/R2020b\"],\"version\":\"1.0\"}"
  "Full Order Observer " : Subsystem
  Full Order Observer Dynamic : Subsystem
  Static Pre-compensator Observer : Subsystem
      settings: PortSchema="{\"entries\":[{\"content\":{\"sides\":[{\"content\":{\"connectorIds\":[\"In1\"]},\"type\":\"ConnectorPlacement.EquallySpacedRectSide\",\"uuid\":\"d610b34c-52eb-4819-8d1a-81d5a985b9d9\"},{\"content\":{\"connectorIds\":[\"Out1\"],\"side\":\"RIGHT\"},\"type\":\"ConnectorPlacement.EquallySpacedRectSide\",\"uuid\":\"fa39cbc5-3568-4c29-bd8a-db3473067912\"},{\"content\":{\"connectorIds\":[\"In2\"],\"side\":\"TOP\"},\"type\":\"ConnectorPlacement.EquallySpacedRectSide\",\"uuid\":\"3b0c7600-722f-4b06-adf0-1b1e252bb733\"}]},\"type\":\"ConnectorPlacement.EquallySpacedConnector\",\"uuid\":\"5ae79dff-d54b-4499-8ef0-57db3eb052a8\"}],\"packageUris\":[\"http://schema.mathworks.com/mf0/Connector/R2020b\"],\"version\":\"1.0\"}"
  US_L : Outport
  x_hat_LS : Outport  Port=2
  UD_L : Outport  Port=3
  x_hat_LD : Outport  Port=4
  wires:
  Full Order Observer Dynamic/1(x_hat_L) -> Dynamic Pre-compensator Observer/1(x_hat_L), x_hat_LD/1
  y/1 -> Full Order Observer Dynamic/2(y_L), Dynamic Pre-compensator Observer/2(y), "Full Order Observer "/1(y_L)
  u/1 -> Static Pre-compensator Observer/2(u), Dynamic Pre-compensator Observer/3(u)
  Dynamic Pre-compensator Observer/1(Linear Sys input) -> Full Order Observer Dynamic/1(u_L - kx), UD_L/1
  Static Pre-compensator Observer/1(Linear Sys input) -> "Full Order Observer "/2(u_L - kx), US_L/1
  "Full Order Observer "/1(x_hat_L) -> x_hat_LS/1, Static Pre-compensator Observer/1(x_hat_L)

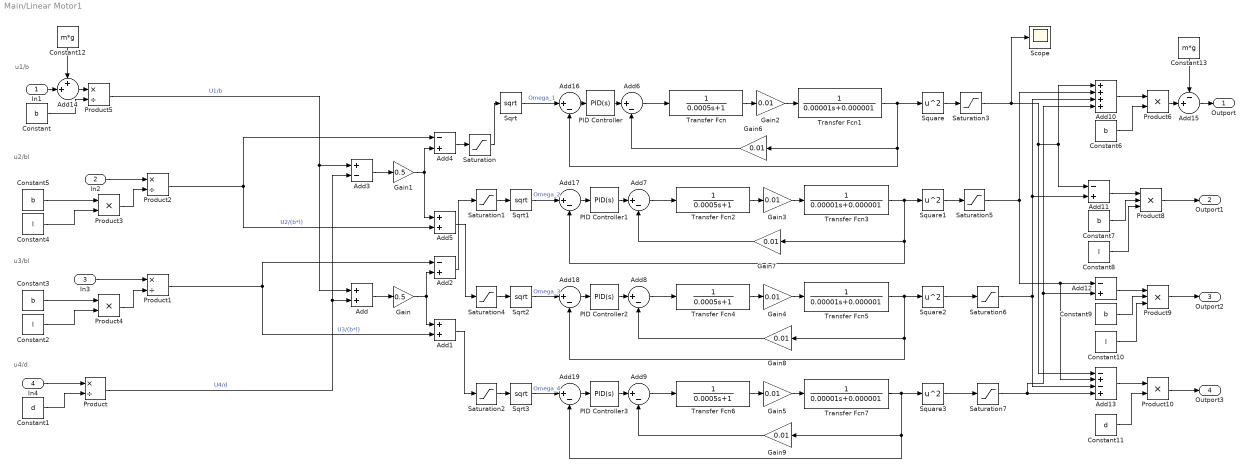
== system Main/Linear Motor1 ==
  note: u1/b
  note: u2/bl
  note: u3/bl
  note: u4/d
  In1 : Inport
  In2 : Inport  Port=2
  In3 : Inport  Port=3
  In4 : Inport  Port=4
  Add : Sum
  Add1 : Sum
  Add10 : Sum  Inputs=++++
  Add{2,4,11..12} (4 alike) : Sum  Inputs=-+
  Add13 : Sum  Inputs=-+-+
  Add14 : Sum  Inputs=++|
  Add15 : Sum  Inputs=-+|
  Add{6..9,16..19} (8 alike) : Sum  Inputs=|+-
  Add3 : Sum  Inputs=+-
  Add5 : Sum
  Constant{,3,5..7,9} (6 alike) : Constant  Value=b
  Constant1 : Constant  Value=d
  Constant{2,4,8,10} (4 alike) : Constant  Value=l
  Constant11 : Constant  Value=d
  Constant12 : Constant  Value=m*g
  Constant13 : Constant  Value=m*g
  Gain : Gain  Gain=0.5
  Gain1 : Gain  Gain=0.5
  Gain{2..9} (8 alike) : Gain  Gain=0.01
  PID Controller{,1..3} (4 alike) : slpidlib/PID Controller  Controller=PID  Form=Parallel  TimeDomain=Continuous-time  UseExternalTs=off  SampleTime=-1  IntegratorMethod=Forward Euler  FilterMethod=Forward Euler  ControllerParametersSource=internal  P=0.171554924473584  I=7.26619368797272  UseKiTs=off  D=0  N=100  UseFilter=on  TunerSelectOption=Transfer Function Based (PID Tuner App)  InitialConditionSource=internal  InitialConditionForIntegrator=0  InitialConditionForFilter=0  DifferentiatorICPrevScaledInput=0  ExternalReset=none  TrackingMode=off  Kt=1  LimitOutput=off  SatLimitsSource=internal  UpperSaturationLimit=inf  LowerSaturationLimit=-inf  LinearizeAsGain=on  AntiWindupMode=none  Kb=1  POutMin=[]  POutMax=[]  IOutMin=[]  IOutMax=[]  DOutMin=[]  DOutMax=[]  NOutMin=[]  NOutMax=[]  SumOutMin=[]  SumOutMax=[]  SaturationOutMin=[]  SaturationOutMax=[]  PParamMin=[]  PParamMax=[]  IParamMin=[]  IParamMax=[]  DParamMin=[]  DParamMax=[]  NParamMin=[]  NParamMax=[]  KbParamMin=[]  KbParamMax=[]  KtParamMin=[]  KtParamMax=[]  KbOutMin=[]  KbOutMax=[]  KtOutMin=[]  KtOutMax=[]  IntegratorOutMin=[]  IntegratorOutMax=[]  FilterOutMin=[]  FilterOutMax=[]  SumI1OutMin=[]  SumI1OutMax=[]  SumI2OutMin=[]  SumI2OutMax=[]  SumI3OutMin=[]  SumI3OutMax=[]  SumI4OutMin=[]  SumI4OutMax=[]  SumDOutMin=[]  SumDOutMax=[]  DifferentiatorOutMin=[]  DifferentiatorOutMax=[]  FilterDiffOutCoefMin=[]  FilterDiffOutCoefMax=[]  ReciprocalOutMin=[]  ReciprocalOutMax=[]  SumDenOutMin=[]  SumDenOutMax=[]  SumNumOutMin=[]  SumNumOutMax=[]  DivideOutMin=[]  DivideOutMax=[]  UdiffTsProdOutMin=[]  UdiffTsProdOutMax=[]  NTsProdOutMin=[]  NTsProdOutMax=[]  UintegralTsProdOutMin=[]  UintegralTsProdOutMax=[]  UngainTsProdOutMin=[]  UngainTsProdOutMax=[]  IntegratorContinuousStateAttributes=''  IntegratorStateMustResolveToSignalObject=off  IntegratorRTWStateStorageClass=Auto  FilterContinuousStateAttributes=''  FilterStateMustResolveToSignalObject=off  FilterRTWStateStorageClass=Auto  ParallelPVariant=InternalParameters  IdealPVariant=Disabled  IVariant=InternalParameters  DVariant=InternalParameters  IntegratorVariant=Continuous  SatVariant=Disabled  AWVariant=Passthrough  PCopyVariant=Disabled  TRVariant=Disabled  FdbkBlocksVariant=Forward  IdealPFdbkVariant=Disabled  SatFdbkVariant=Disabled  DerivativeFilterVariant=ContFilter  NVariant=InternalParameters  NCopyVariant=Disabled  FilterICVariant=InternalICsFilter  IntegratorICVariant=InternalICs  ExternalResetVariant=Disabled  TRSumVariant=Passthrough  SumFdbkVariant=Disabled  SumVariant=Sum_PID  TsampFilterVariant=InternalTs  TsampNgainVariant=Passthrough  TsampIntegralVariant=Passthrough  ExternalSaturationOutDataTypeStr=Inherit: Same as second input
  Product{,1..2,5} (4 alike) : Product  Inputs=*/
  Product{3..4,6,10} (4 alike) : Product
  Product8 : Product  Inputs=3
  Product9 : Product  Inputs=3
  Saturation{,1..7} (8 alike) : Saturate  UpperLimit=82000  LowerLimit=0
  Scope : Scope
  Sqrt{,1..3} (4 alike) : Sqrt
  Square{,1..3} (4 alike) : Math  Operator=square
  Transfer Fcn{,2,4,6} (4 alike) : TransferFcn  Denominator=[0.0005 1]
  Transfer Fcn{1,3,5,7} (4 alike) : TransferFcn  Denominator=[0.00001 0.000001]
  Outport : Outport
  Outport1 : Outport  Port=2
  Outport2 : Outport  Port=3
  Outport3 : Outport  Port=4
  wires:
  In4/1 -> Product/1
  Constant1/1 -> Product/2
  Product4/1 -> Product1/2
  Constant2/1 -> Product4/2
  In3/1 -> Product1/1
  Constant3/1 -> Product4/1
  Product3/1 -> Product2/2
  Constant4/1 -> Product3/2
  In2/1 -> Product2/1
  Constant5/1 -> Product3/1
  Constant/1 -> Product5/2
  Product5/1 -> Add3/1, Add/1  "U1/b"
  Product/1 -> Add3/2, Add/2  "U4/d"
  Add/1 -> Gain/1
  Gain/1 -> Add1/1, Add2/2
  Product1/1 -> Add1/2, Add2/1  "U3/(b*l)"
  Add3/1 -> Gain1/1
  Gain1/1 -> Add5/1, Add4/2
  Product2/1 -> Add5/2, Add4/1  "U2/(b*l)"
  Transfer Fcn/1 -> Gain2/1
  Gain2/1 -> Transfer Fcn1/1
  Add6/1 -> Transfer Fcn/1
  Transfer Fcn2/1 -> Gain3/1
  Transfer Fcn3/1 -> Gain7/1, Add17/2, Square1/1
  Add7/1 -> Transfer Fcn2/1
  Gain3/1 -> Transfer Fcn3/1
  Add8/1 -> Transfer Fcn4/1
  Gain4/1 -> Transfer Fcn5/1
  Transfer Fcn4/1 -> Gain4/1
  Transfer Fcn5/1 -> Gain8/1, Add18/2, Square2/1
  Add9/1 -> Transfer Fcn6/1
  Gain5/1 -> Transfer Fcn7/1
  Transfer Fcn6/1 -> Gain5/1
  Transfer Fcn7/1 -> Gain9/1, Add19/2, Square3/1
  Transfer Fcn1/1 -> Add16/2, Gain6/1, Square/1
  Square/1 -> Saturation3/1
  Square1/1 -> Saturation5/1
  Square2/1 -> Saturation6/1
  Square3/1 -> Saturation7/1
  Add10/1 -> Product6/1
  Constant6/1 -> Product6/2
  Add11/1 -> Product8/1
  Constant7/1 -> Product8/2
  Constant8/1 -> Product8/3
  Add12/1 -> Product9/1
  Constant9/1 -> Product9/2
  Constant10/1 -> Product9/3
  Add13/1 -> Product10/1
  Constant11/1 -> Product10/2
  Product8/1 -> Outport1/1
  Product9/1 -> Outport2/1
  Product10/1 -> Outport3/1
  Gain6/1 -> Add6/2
  Gain7/1 -> Add7/2
  Gain8/1 -> Add8/2
  Gain9/1 -> Add9/2
  Add4/1 -> Saturation/1
  Add2/1 -> Saturation1/1
  Add5/1 -> Saturation4/1
  Add1/1 -> Saturation2/1
  Saturation/1 -> Sqrt/1
  Saturation1/1 -> Sqrt1/1
  Saturation4/1 -> Sqrt2/1
  Saturation2/1 -> Sqrt3/1
  Saturation3/1 -> Scope/1, Add13/1, Add11/1, Add10/1
  Saturation5/1 -> Add13/2, Add12/1, Add10/2
  Saturation6/1 -> Add13/3, Add11/2, Add10/3
  Saturation7/1 -> Add12/2, Add10/4, Add13/4
  In1/1 -> Add14/2
  Add14/1 -> Product5/1
  Constant12/1 -> Add14/1
  Sqrt/1 -> Add16/1  "Omega_1"
  Add16/1 -> PID Controller/1
  PID Controller/1 -> Add6/1
  Sqrt1/1 -> Add17/1  "Omega_2"
  Add17/1 -> PID Controller1/1
  PID Controller1/1 -> Add7/1
  Sqrt2/1 -> Add18/1  "Omega_3"
  Add18/1 -> PID Controller2/1
  PID Controller2/1 -> Add8/1
  Sqrt3/1 -> Add19/1  "Omega_4"
  Add19/1 -> PID Controller3/1
  PID Controller3/1 -> Add9/1
  Constant13/1 -> Add15/1
  Product6/1 -> Add15/2
  Add15/1 -> Outport/1

== system Main/MAE Observer ==
  x : Inport
  x_hat : Inport  Port=2
  Time : Inport  Port=3
  Enable : EnablePort
  Abs : Abs  SaturateOnIntegerOverflow=off
  Add7 : Sum  Inputs=+-
  Display1 : Display
  Divide : Product  Inputs=*/
  Integrator : Integrator
  MAE : Outport
  wires:
  x/1 -> Add7/1
  Add7/1 -> Abs/1
  Divide/1 -> Display1/1, MAE/1
  Integrator/1 -> Divide/1
  Time/1 -> Divide/2
  x_hat/1 -> Add7/2
  Abs/1 -> Integrator/1

== system Main/MAE Trajectory ==
  u : Inport
  y : Inport  Port=2
  Time : Inport  Port=3
  Enable : EnablePort
  Abs : Abs  SaturateOnIntegerOverflow=off
  Add7 : Sum  Inputs=+-
  Display1 : Display
  Divide : Product  Inputs=*/
  Integrator : Integrator
  MAE : Outport
  wires:
  u/1 -> Add7/1
  Add7/1 -> Abs/1
  Divide/1 -> Display1/1, MAE/1
  Integrator/1 -> Divide/1
  Time/1 -> Divide/2
  y/1 -> Add7/2
  Abs/1 -> Integrator/1

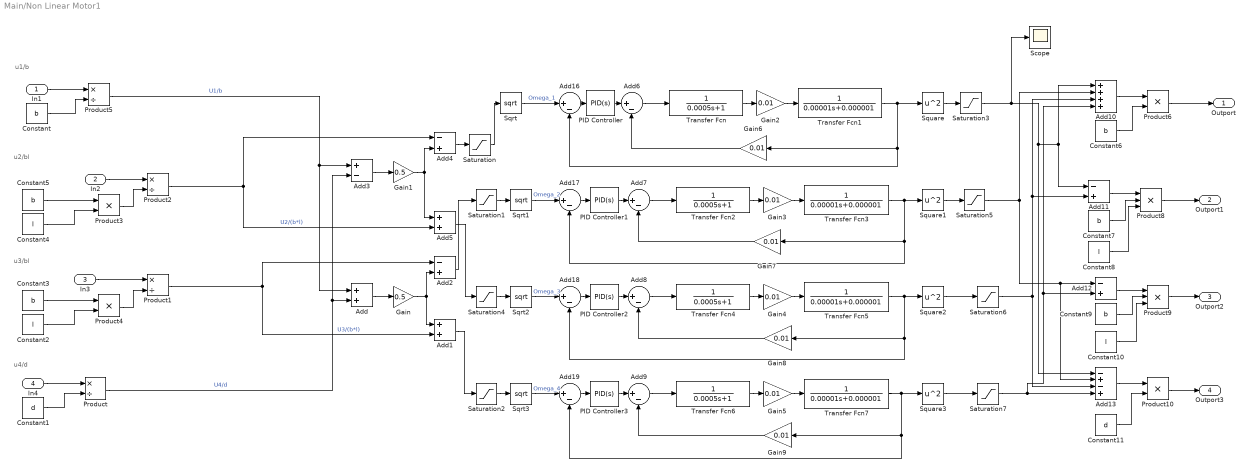
== system Main/Non Linear Motor1 ==
  note: u1/b
  note: u2/bl
  note: u3/bl
  note: u4/d
  In1 : Inport
  In2 : Inport  Port=2
  In3 : Inport  Port=3
  In4 : Inport  Port=4
  Add : Sum
  Add1 : Sum
  Add10 : Sum  Inputs=++++
  Add{2,4,11..12} (4 alike) : Sum  Inputs=-+
  Add13 : Sum  Inputs=-+-+
  Add{6..9,16..19} (8 alike) : Sum  Inputs=|+-
  Add3 : Sum  Inputs=+-
  Add5 : Sum
  Constant{,3,5..7,9} (6 alike) : Constant  Value=b
  Constant1 : Constant  Value=d
  Constant{2,4,8,10} (4 alike) : Constant  Value=l
  Constant11 : Constant  Value=d
  Gain : Gain  Gain=0.5
  Gain1 : Gain  Gain=0.5
  Gain{2..9} (8 alike) : Gain  Gain=0.01
  PID Controller{,1..3} (4 alike) : slpidlib/PID Controller  Controller=PID  Form=Parallel  TimeDomain=Continuous-time  UseExternalTs=off  SampleTime=-1  IntegratorMethod=Forward Euler  FilterMethod=Forward Euler  ControllerParametersSource=internal  P=0.171554924473584  I=7.26619368797272  UseKiTs=off  D=0  N=100  UseFilter=on  TunerSelectOption=Transfer Function Based (PID Tuner App)  InitialConditionSource=internal  InitialConditionForIntegrator=0  InitialConditionForFilter=0  DifferentiatorICPrevScaledInput=0  ExternalReset=none  TrackingMode=off  Kt=1  LimitOutput=off  SatLimitsSource=internal  UpperSaturationLimit=inf  LowerSaturationLimit=-inf  LinearizeAsGain=on  AntiWindupMode=none  Kb=1  POutMin=[]  POutMax=[]  IOutMin=[]  IOutMax=[]  DOutMin=[]  DOutMax=[]  NOutMin=[]  NOutMax=[]  SumOutMin=[]  SumOutMax=[]  SaturationOutMin=[]  SaturationOutMax=[]  PParamMin=[]  PParamMax=[]  IParamMin=[]  IParamMax=[]  DParamMin=[]  DParamMax=[]  NParamMin=[]  NParamMax=[]  KbParamMin=[]  KbParamMax=[]  KtParamMin=[]  KtParamMax=[]  KbOutMin=[]  KbOutMax=[]  KtOutMin=[]  KtOutMax=[]  IntegratorOutMin=[]  IntegratorOutMax=[]  FilterOutMin=[]  FilterOutMax=[]  SumI1OutMin=[]  SumI1OutMax=[]  SumI2OutMin=[]  SumI2OutMax=[]  SumI3OutMin=[]  SumI3OutMax=[]  SumI4OutMin=[]  SumI4OutMax=[]  SumDOutMin=[]  SumDOutMax=[]  DifferentiatorOutMin=[]  DifferentiatorOutMax=[]  FilterDiffOutCoefMin=[]  FilterDiffOutCoefMax=[]  ReciprocalOutMin=[]  ReciprocalOutMax=[]  SumDenOutMin=[]  SumDenOutMax=[]  SumNumOutMin=[]  SumNumOutMax=[]  DivideOutMin=[]  DivideOutMax=[]  UdiffTsProdOutMin=[]  UdiffTsProdOutMax=[]  NTsProdOutMin=[]  NTsProdOutMax=[]  UintegralTsProdOutMin=[]  UintegralTsProdOutMax=[]  UngainTsProdOutMin=[]  UngainTsProdOutMax=[]  IntegratorContinuousStateAttributes=''  IntegratorStateMustResolveToSignalObject=off  IntegratorRTWStateStorageClass=Auto  FilterContinuousStateAttributes=''  FilterStateMustResolveToSignalObject=off  FilterRTWStateStorageClass=Auto  ParallelPVariant=InternalParameters  IdealPVariant=Disabled  IVariant=InternalParameters  DVariant=InternalParameters  IntegratorVariant=Continuous  SatVariant=Disabled  AWVariant=Passthrough  PCopyVariant=Disabled  TRVariant=Disabled  FdbkBlocksVariant=Forward  IdealPFdbkVariant=Disabled  SatFdbkVariant=Disabled  DerivativeFilterVariant=ContFilter  NVariant=InternalParameters  NCopyVariant=Disabled  FilterICVariant=InternalICsFilter  IntegratorICVariant=InternalICs  ExternalResetVariant=Disabled  TRSumVariant=Passthrough  SumFdbkVariant=Disabled  SumVariant=Sum_PID  TsampFilterVariant=InternalTs  TsampNgainVariant=Passthrough  TsampIntegralVariant=Passthrough  ExternalSaturationOutDataTypeStr=Inherit: Same as second input
  Product{,1..2,5} (4 alike) : Product  Inputs=*/
  Product{3..4,6,10} (4 alike) : Product
  Product8 : Product  Inputs=3
  Product9 : Product  Inputs=3
  Saturation{,1..7} (8 alike) : Saturate  UpperLimit=82000  LowerLimit=0
  Scope : Scope
  Sqrt{,1..3} (4 alike) : Sqrt
  Square{,1..3} (4 alike) : Math  Operator=square
  Transfer Fcn{,2,4,6} (4 alike) : TransferFcn  Denominator=[0.0005 1]
  Transfer Fcn{1,3,5,7} (4 alike) : TransferFcn  Denominator=[0.00001 0.000001]
  Outport : Outport
  Outport1 : Outport  Port=2
  Outport2 : Outport  Port=3
  Outport3 : Outport  Port=4
  wires:
  In4/1 -> Product/1
  Constant1/1 -> Product/2
  Product4/1 -> Product1/2
  Constant2/1 -> Product4/2
  In3/1 -> Product1/1
  Constant3/1 -> Product4/1
  Product3/1 -> Product2/2
  Constant4/1 -> Product3/2
  In2/1 -> Product2/1
  Constant5/1 -> Product3/1
  Constant/1 -> Product5/2
  Product5/1 -> Add3/1, Add/1  "U1/b"
  Product/1 -> Add3/2, Add/2  "U4/d"
  Add/1 -> Gain/1
  Gain/1 -> Add1/1, Add2/2
  Product1/1 -> Add1/2, Add2/1  "U3/(b*l)"
  Add3/1 -> Gain1/1
  Gain1/1 -> Add5/1, Add4/2
  Product2/1 -> Add5/2, Add4/1  "U2/(b*l)"
  Transfer Fcn/1 -> Gain2/1
  Gain2/1 -> Transfer Fcn1/1
  Add6/1 -> Transfer Fcn/1
  Transfer Fcn2/1 -> Gain3/1
  Transfer Fcn3/1 -> Gain7/1, Add17/2, Square1/1
  Add7/1 -> Transfer Fcn2/1
  Gain3/1 -> Transfer Fcn3/1
  Add8/1 -> Transfer Fcn4/1
  Gain4/1 -> Transfer Fcn5/1
  Transfer Fcn4/1 -> Gain4/1
  Transfer Fcn5/1 -> Gain8/1, Add18/2, Square2/1
  Add9/1 -> Transfer Fcn6/1
  Gain5/1 -> Transfer Fcn7/1
  Transfer Fcn6/1 -> Gain5/1
  Transfer Fcn7/1 -> Gain9/1, Add19/2, Square3/1
  Transfer Fcn1/1 -> Add16/2, Gain6/1, Square/1
  Square/1 -> Saturation3/1
  Square1/1 -> Saturation5/1
  Square2/1 -> Saturation6/1
  Square3/1 -> Saturation7/1
  Add10/1 -> Product6/1
  Constant6/1 -> Product6/2
  Add11/1 -> Product8/1
  Constant7/1 -> Product8/2
  Constant8/1 -> Product8/3
  Add12/1 -> Product9/1
  Constant9/1 -> Product9/2
  Constant10/1 -> Product9/3
  Add13/1 -> Product10/1
  Constant11/1 -> Product10/2
  Product8/1 -> Outport1/1
  Product9/1 -> Outport2/1
  Product10/1 -> Outport3/1
  Gain6/1 -> Add6/2
  Gain7/1 -> Add7/2
  Gain8/1 -> Add8/2
  Gain9/1 -> Add9/2
  Add4/1 -> Saturation/1
  Add2/1 -> Saturation1/1
  Add5/1 -> Saturation4/1
  Add1/1 -> Saturation2/1
  Saturation/1 -> Sqrt/1
  Saturation1/1 -> Sqrt1/1
  Saturation4/1 -> Sqrt2/1
  Saturation2/1 -> Sqrt3/1
  Saturation3/1 -> Scope/1, Add13/1, Add11/1, Add10/1
  Saturation5/1 -> Add13/2, Add12/1, Add10/2
  Saturation6/1 -> Add13/3, Add11/2, Add10/3
  Saturation7/1 -> Add12/2, Add10/4, Add13/4
  In1/1 -> Product5/1
  Sqrt/1 -> Add16/1  "Omega_1"
  Add16/1 -> PID Controller/1
  PID Controller/1 -> Add6/1
  Sqrt1/1 -> Add17/1  "Omega_2"
  Add17/1 -> PID Controller1/1
  PID Controller1/1 -> Add7/1
  Sqrt2/1 -> Add18/1  "Omega_3"
  Add18/1 -> PID Controller2/1
  PID Controller2/1 -> Add8/1
  Sqrt3/1 -> Add19/1  "Omega_4"
  Add19/1 -> PID Controller3/1
  PID Controller3/1 -> Add9/1
  Product6/1 -> Outport/1

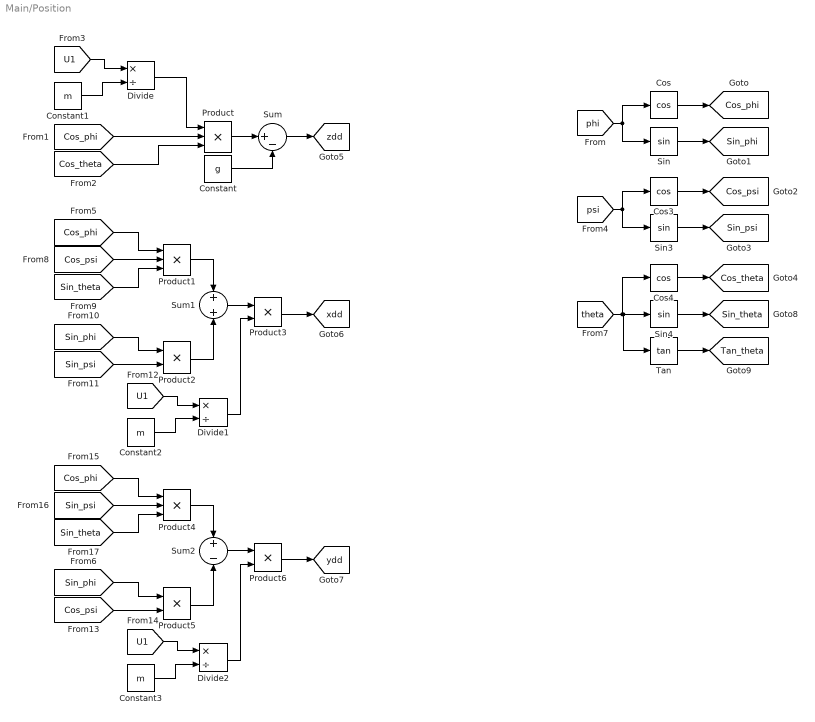
== system Main/Position ==
  Constant : Constant  Value=g
  Constant1 : Constant  Value=m
  Constant2 : Constant  Value=m
  Constant3 : Constant  Value=m
  Cos : Trigonometry  Operator=cos
  Cos3 : Trigonometry  Operator=cos
  Cos4 : Trigonometry  Operator=cos
  Divide : Product  Inputs=*/
  Divide1 : Product  Inputs=*/
  Divide2 : Product  Inputs=*/
  Product : Product  Inputs=3
  Product1 : Product  Inputs=3
  Product{2..3,5..6} (4 alike) : Product
  Product4 : Product  Inputs=3
  Sin : Trigonometry
  Sin3 : Trigonometry
  Sin4 : Trigonometry
  Sum : Sum  Inputs=|+-
  Sum1 : Sum
  Sum2 : Sum  Inputs=+-
  Tan : Trigonometry  Operator=tan
  tag scope: Cos_phi=global, Cos_psi=global, Cos_theta=global, Sin_phi=global, Sin_psi=global, Sin_theta=global, Tan_theta=global, xdd=global, ydd=global, zdd=global
  wires:
  Constant/1 -> Sum/2
  Product/1 -> Sum/1
  Sum/1 -> [zdd]
  Constant1/1 -> Divide/2
  [U1] -> Divide/1
  Divide/1 -> Product/1
  [phi] -> Cos/1, Sin/1
  Cos/1 -> [Cos_phi]
  Sin/1 -> [Sin_phi]
  Sin3/1 -> [Sin_psi]
  Cos3/1 -> [Cos_psi]
  [psi] -> Cos3/1, Sin3/1
  Sin4/1 -> [Sin_theta]
  Cos4/1 -> [Cos_theta]
  [theta] -> Cos4/1, Tan/1, Sin4/1
  [Cos_phi] -> Product/2
  [Cos_theta] -> Product/3
  [Cos_phi] -> Product1/1
  [Cos_psi] -> Product1/2
  [Sin_theta] -> Product1/3
  [Sin_psi] -> Product2/2
  [Sin_phi] -> Product2/1
  Product2/1 -> Sum1/2
  Product1/1 -> Sum1/1
  Product3/1 -> [xdd]
  Sum1/1 -> Product3/1
  Constant2/1 -> Divide1/2
  [U1] -> Divide1/1
  Divide1/1 -> Product3/2
  Product4/1 -> Sum2/1
  [Sin_theta] -> Product4/3
  Constant3/1 -> Divide2/2
  [Sin_psi] -> Product4/2
  [Cos_phi] -> Product4/1
  Product5/1 -> Sum2/2
  Divide2/1 -> Product6/2
  Sum2/1 -> Product6/1
  [Sin_phi] -> Product5/1
  [U1] -> Divide2/1
  [Cos_psi] -> Product5/2
  Product6/1 -> [ydd]
  Tan/1 -> [Tan_theta]

== system Main/Reduced Order Observer ==
  note: Reduced Oreder Observer
  y : Inport
  u : Inport  Port=2
  Dynamic Pre-compensator : Subsystem
      settings: PortSchema="{\"entries\":[{\"content\":{\"sides\":[{\"content\":{\"connectorIds\":[\"In1\"]},\"type\":\"ConnectorPlacement.EquallySpacedRectSide\",\"uuid\":\"41f0ab22-05fc-4f3b-83bb-0a50654efd65\"},{\"content\":{\"connectorIds\":[\"Out1\"],\"side\":\"RIGHT\"},\"type\":\"ConnectorPlacement.EquallySpacedRectSide\",\"uuid\":\"0f7ef9da-8381-47a4-9bca-562d92f17fdf\"},{\"content\":{\"connectorIds\":[\"In2\",\"In3\"],\"side\":\"TOP\"},\"type\":\"ConnectorPlacement.EquallySpacedRectSide\",\"uuid\":\"cd81a1c1-f0e3-4bb0-80bc-d77bdf86c649\"}]},\"type\":\"ConnectorPlacement.EquallySpacedConnector\",\"uuid\":\"0ac9f9f6-6bd1-43d5-a807-6300901c238f\"}],\"packageUris\":[\"http://schema.mathworks.com/mf0/Connector/R2020b\"],\"version\":\"1.0\"}"
  Full Order Observer Reduced Static : Subsystem
  Full Order Observer Reduced Static1 : Subsystem
  Static Pre-compensator Reduced Observer : Subsystem
      settings: PortSchema="{\"entries\":[{\"content\":{\"sides\":[{\"content\":{\"connectorIds\":[\"In1\"]},\"type\":\"ConnectorPlacement.EquallySpacedRectSide\",\"uuid\":\"d610b34c-52eb-4819-8d1a-81d5a985b9d9\"},{\"content\":{\"connectorIds\":[\"Out1\"],\"side\":\"RIGHT\"},\"type\":\"ConnectorPlacement.EquallySpacedRectSide\",\"uuid\":\"fa39cbc5-3568-4c29-bd8a-db3473067912\"},{\"content\":{\"connectorIds\":[],\"side\":\"TOP\"},\"type\":\"ConnectorPlacement.EquallySpacedRectSide\",\"uuid\":\"3b0c7600-722f-4b06-adf0-1b1e252bb733\"},{\"content\":{\"connectorIds\":[\"In2\"],\"side\":\"BOTTOM\"},\"type\":\"ConnectorPlacement.EquallySpacedRectSide\",\"uuid\":\"cad8b764-58a3-4ada-a672-9e0aa7c39766\"}]},\"type\":\"ConnectorPlacement.EquallySpacedConnector\",\"uuid\":\"5ae79dff-d54b-4499-8ef0-57db3eb052a8\"}],\"packageUris\":[\"http://schema.mathworks.com/mf0/Connector/R2020b\"],\"version\":\"1.0\"}"
  US_L : Outport
  x_hat_DS : Outport  Port=2
  UD_L : Outport  Port=3
  x_hat_LS : Outport  Port=4
  wires:
  Static Pre-compensator Reduced Observer/1(Linear Sys input) -> US_L/1, Full Order Observer Reduced Static/1(u_L - kx)
  u/1 -> Static Pre-compensator Reduced Observer/2(u), Dynamic Pre-compensator/3(u)
  Full Order Observer Reduced Static/1(x_hat_reduced) -> x_hat_DS/1, Static Pre-compensator Reduced Observer/1(x_hat_L)
  y/1 -> Dynamic Pre-compensator/2(y), Full Order Observer Reduced Static/2(y_L), Full Order Observer Reduced Static1/1(y_L)
  Full Order Observer Reduced Static1/1(x_hat_reduced) -> x_hat_LS/1, Dynamic Pre-compensator/1(x_hat_L)
  Dynamic Pre-compensator/1(Linear Sys input) -> UD_L/1, Full Order Observer Reduced Static1/2(u_L - kx)

== system Main/Static Pre-compensator ==
  Trajectory : Inport
  Add1 : Sum  Inputs=-+
  Add3 : Sum  Inputs=-+
  Matrix Multiply{,1..3} (4 alike) : Product  Multiplication=Matrix(*)
  Non linear Sys input : Outport
  Linear Sys input : Outport  Port=2
  wires:
  Matrix Multiply1/1 -> Add3/1
  [States] -> Matrix Multiply1/2
  [K_State] -> Matrix Multiply1/1
  Add3/1 -> Non linear Sys input/1
  Matrix Multiply2/1 -> Add3/2
  [Gain_Static] -> Matrix Multiply2/1
  Matrix Multiply/1 -> Add1/1
  [X_linear] -> Matrix Multiply/2
  [K_State] -> Matrix Multiply/1
  Trajectory/1 -> Matrix Multiply3/2, Matrix Multiply2/2
  Matrix Multiply3/1 -> Add1/2
  [Gain_Static] -> Matrix Multiply3/1
  Add1/1 -> Linear Sys input/1
